simulink model "VectorTrackingSim"  (R2023a)
settings: Solver=FixedStepAuto  StartTime=Start_Time  StopTime=End_Time  FixedStep=Time_Step  RelTol=1e-3
values from neighbouring files (symbols this model uses):
  BSFC_LUT = aircraft.BSFC_LUT    [FVDM_Noise.m]    (also in FVDM_Truth.m)
  STGeometry = aircraft.STGeometry    [FVDM_Noise.m]    (also in FVDM_Truth.m)
  Vehicle = aircraft.Vehicle    [FVDM_Noise.m]    (also in FVDM_Truth.m)
undefined symbols (not defined in the file or in its folder): dayofyear, Earth, Initial_X, lookaheadDist, PowerFactor_LUT, waypoints, WGS84
libraries: slpidlib x7, simulink_extras x3, aerolibtransform2 x1, aerolibatmos2 x1, uavalgslib x1
(part 1 of 2)
settings Model: Creator=izc0018  LastModifiedBy=noahm
settings DebuggingCC: AlgebraicLoopMsg=none  UnconnectedInputMsg=warning  UnconnectedOutputMsg=warning  UnconnectedLineMsg=warning
settings HardwareCC: ProdBitPerLong=64  ProdLargestAtomicFloat=None  ProdHWDeviceType=AMD->Athlon 64
settings ModelReferenceCC: EnableRefExpFcnMdlSchedulingChecks=on  ModelReferenceMinAlgLoopOccurrences=on
settings RTWCC: DLArmComputeVersion=19.05

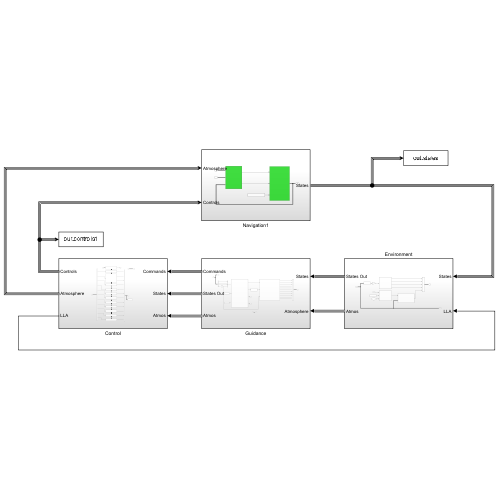
[thumbnail: Simulink's stored preview of the top-level diagram]
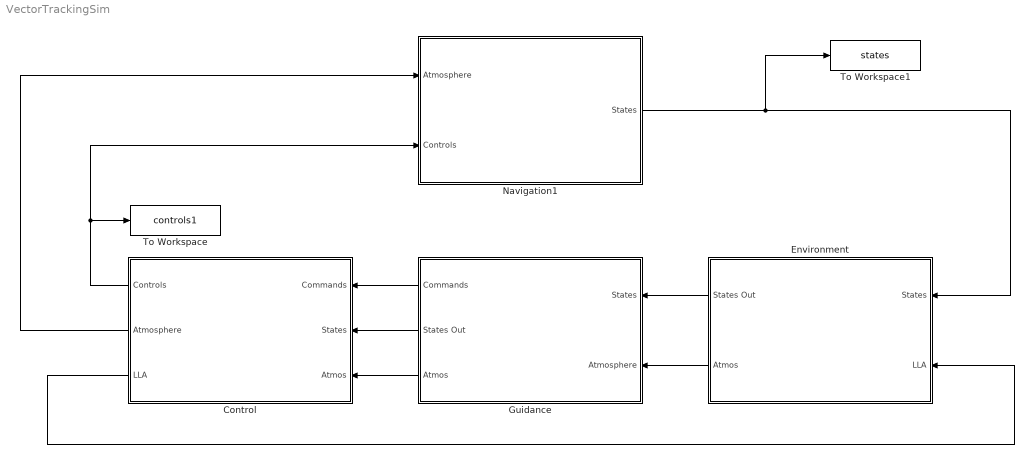
== system VectorTrackingSim ==
  Control : Subsystem
  Environment : Subsystem
  Guidance : Subsystem
  Navigation1 : Subsystem
  To Workspace : ToWorkspace  VariableName=controls1  SampleTime=-1
      settings: Save2DSignal=2-D array (concatenate along first dimension)
  To Workspace1 : ToWorkspace  VariableName=states  SampleTime=-1
      settings: Save2DSignal=2-D array (concatenate along first dimension)
  wires:
  Control/2(Atmosphere) -> Navigation1/1(Atmosphere)
  Guidance/1(Commands) -> Control/1(Commands)
  Environment/2(Atmos) -> Guidance/2(Atmosphere)
  Navigation1/1(States) -> To Workspace1/1, Environment/1(States)
  Control/3(LLA) -> Environment/2(LLA)
  Guidance/2(States Out) -> Control/2(States)
  Guidance/3(Atmos) -> Control/3(Atmos)
  Control/1(Controls) -> Navigation1/2(Controls), To Workspace/1
  Environment/1(States Out) -> Guidance/1(States)

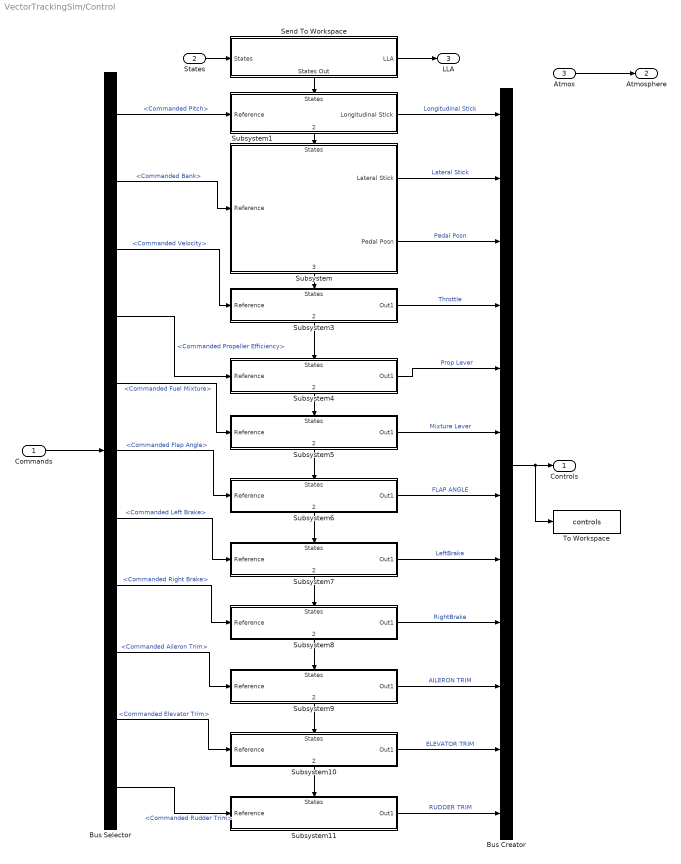
== system VectorTrackingSim/Control ==
  Commands : Inport
  States : Inport  Port=2
  Atmos : Inport  Port=3
  Bus Creator : BusCreator  Inputs=12
  Bus Selector : BusSelector  OutputSignals=Commanded Pitch,Commanded Bank,Commanded Velocity,Commanded Propeller Efficiency,Commanded Fuel Mixture,Commanded Flap Angle,Commanded Left Brake,Commanded Right Brake,Commanded Aileron Trim,Commanded Elevator Trim,Commanded Rudder Trim
  Send To Workspace : Subsystem
      settings: PortSchema="{\"entries\":[{\"content\":{\"sides\":[{\"content\":{\"connectorIds\":[\"In1\"]},\"type\":\"ConnectorPlacement.EquallySpacedRectSide\",\"uuid\":\"f8d70518-feba-4467-9144-e72499141e10\"},{\"content\":{\"connectorIds\":[\"Out1\"],\"side\":\"RIGHT\"},\"type\":\"ConnectorPlacement.EquallySpacedRectSide\",\"uuid\":\"0d837ca8-6650-40ee-933a-3521e14176de\"},{\"content\":{\"side\":\"TOP\"},\"type\":\"ConnectorPlacement.EquallySpacedRectSide\",\"uuid\":\"54f7b60b-7724-46f0-8f38-219401d515c7\"},{\"content\":{\"connectorIds\":[\"Out2\"],\"side\":\"BOTTOM\"},\"type\":\"ConnectorPlacement.EquallySpacedRectSide\",\"uuid\":\"f1e71b5c-4796-4085-9245-75f71ccb39d6\"}]},\"type\":\"ConnectorPlacement.EquallySpacedConnector\",\"uuid\":\"946e06f8-2adb-45c5-9153-0b4b2f8d0bb6\"}],\"packageUris\":[\"http://schema.mathworks.com/mf0/Connector/R2020b\"],\"version\":\"1.0\"}"
  Subsystem : Subsystem
      settings: PortSchema="{\"entries\":[{\"content\":{\"sides\":[{\"content\":{\"connectorIds\":[\"In1\"]},\"type\":\"ConnectorPlacement.EquallySpacedRectSide\",\"uuid\":\"5ea7349d-baf6-49c5-809d-4b912ce56d76\"},{\"content\":{\"connectorIds\":[\"Out1\",\"Out2\"],\"side\":\"RIGHT\"},\"type\":\"ConnectorPlacement.EquallySpacedRectSide\",\"uuid\":\"ab3ceec7-e245-42b0-9eb8-e3a68951e219\"},{\"content\":{\"connectorIds\":[\"In2\"],\"side\":\"TOP\"},\"type\":\"ConnectorPlacement.EquallySpacedRectSide\",\"uuid\":\"18178c43-0035-4aec-a3ba-011af3830f5c\"},{\"content\":{\"connectorIds\":[\"Out3\"],\"side\":\"BOTTOM\"},\"type\":\"ConnectorPlacement.EquallySpacedRectSide\",\"uuid\":\"88476787-2df8-4308-98f2-16231590cef9\"}]},\"type\":\"ConnectorPlacement.EquallySpacedConnector\",\"uuid\":\"0f7476f8-a4e6-4d2f-9698-249fd1b1cc90\"}],\"packageUris\":[\"http://schema.mathworks.com/mf0/Connector/R2020b\"],\"version\":\"1.0\"}"
  Subsystem1 : Subsystem
      settings: PortSchema="{\"entries\":[{\"content\":{\"sides\":[{\"content\":{\"connectorIds\":[\"In1\"]},\"type\":\"ConnectorPlacement.EquallySpacedRectSide\",\"uuid\":\"df1e81ab-d97f-43f0-8cd1-ba06c25288e8\"},{\"content\":{\"connectorIds\":[\"Out1\"],\"side\":\"RIGHT\"},\"type\":\"ConnectorPlacement.EquallySpacedRectSide\",\"uuid\":\"fe7f65be-8a13-42ab-8ffa-afe418a633fa\"},{\"content\":{\"connectorIds\":[\"In2\"],\"side\":\"TOP\"},\"type\":\"ConnectorPlacement.EquallySpacedRectSide\",\"uuid\":\"4762097a-1dfd-4646-aeb3-678774417eb9\"},{\"content\":{\"connectorIds\":[\"Out2\"],\"side\":\"BOTTOM\"},\"type\":\"ConnectorPlacement.EquallySpacedRectSide\",\"uuid\":\"338e28fc-4594-4f48-8379-f1c16de78061\"}]},\"type\":\"ConnectorPlacement.EquallySpacedConnector\",\"uuid\":\"e1e6a329-5243-44ef-b6a4-a2802fff17f2\"}],\"packageUris\":[\"http://schema.mathworks.com/mf0/Connector/R2020b\"],\"version\":\"1.0\"}"
  Subsystem10 : Subsystem
      settings: PortSchema="{\"entries\":[{\"content\":{\"sides\":[{\"content\":{\"connectorIds\":[\"In1\"]},\"type\":\"ConnectorPlacement.EquallySpacedRectSide\",\"uuid\":\"df1e81ab-d97f-43f0-8cd1-ba06c25288e8\"},{\"content\":{\"connectorIds\":[\"Out1\"],\"side\":\"RIGHT\"},\"type\":\"ConnectorPlacement.EquallySpacedRectSide\",\"uuid\":\"fe7f65be-8a13-42ab-8ffa-afe418a633fa\"},{\"content\":{\"connectorIds\":[\"In2\"],\"side\":\"TOP\"},\"type\":\"ConnectorPlacement.EquallySpacedRectSide\",\"uuid\":\"4762097a-1dfd-4646-aeb3-678774417eb9\"},{\"content\":{\"connectorIds\":[\"Out2\"],\"side\":\"BOTTOM\"},\"type\":\"ConnectorPlacement.EquallySpacedRectSide\",\"uuid\":\"ca232b1a-28ac-4e7a-b8a6-76103b2c6113\"}]},\"type\":\"ConnectorPlacement.EquallySpacedConnector\",\"uuid\":\"e1e6a329-5243-44ef-b6a4-a2802fff17f2\"}],\"packageUris\":[\"http://schema.mathworks.com/mf0/Connector/R2020b\"],\"version\":\"1.0\"}"
  Subsystem11 : Subsystem
      settings: PortSchema="{\"entries\":[{\"content\":{\"sides\":[{\"content\":{\"connectorIds\":[\"In1\"]},\"type\":\"ConnectorPlacement.EquallySpacedRectSide\",\"uuid\":\"df1e81ab-d97f-43f0-8cd1-ba06c25288e8\"},{\"content\":{\"connectorIds\":[\"Out1\"],\"side\":\"RIGHT\"},\"type\":\"ConnectorPlacement.EquallySpacedRectSide\",\"uuid\":\"fe7f65be-8a13-42ab-8ffa-afe418a633fa\"},{\"content\":{\"connectorIds\":[\"In2\"],\"side\":\"TOP\"},\"type\":\"ConnectorPlacement.EquallySpacedRectSide\",\"uuid\":\"4762097a-1dfd-4646-aeb3-678774417eb9\"}]},\"type\":\"ConnectorPlacement.EquallySpacedConnector\",\"uuid\":\"e1e6a329-5243-44ef-b6a4-a2802fff17f2\"}],\"packageUris\":[\"http://schema.mathworks.com/mf0/Connector/R2020b\"],\"version\":\"1.0\"}"
  Subsystem3 : Subsystem
      settings: PortSchema="{\"entries\":[{\"content\":{\"sides\":[{\"content\":{\"connectorIds\":[\"In1\"]},\"type\":\"ConnectorPlacement.EquallySpacedRectSide\",\"uuid\":\"df1e81ab-d97f-43f0-8cd1-ba06c25288e8\"},{\"content\":{\"connectorIds\":[\"Out1\"],\"side\":\"RIGHT\"},\"type\":\"ConnectorPlacement.EquallySpacedRectSide\",\"uuid\":\"fe7f65be-8a13-42ab-8ffa-afe418a633fa\"},{\"content\":{\"connectorIds\":[\"In2\"],\"side\":\"TOP\"},\"type\":\"ConnectorPlacement.EquallySpacedRectSide\",\"uuid\":\"4762097a-1dfd-4646-aeb3-678774417eb9\"},{\"content\":{\"connectorIds\":[\"Out2\"],\"side\":\"BOTTOM\"},\"type\":\"ConnectorPlacement.EquallySpacedRectSide\",\"uuid\":\"eb7acd08-7b98-4b28-a61a-3ca4385205ec\"}]},\"type\":\"ConnectorPlacement.EquallySpacedConnector\",\"uuid\":\"e1e6a329-5243-44ef-b6a4-a2802fff17f2\"}],\"packageUris\":[\"http://schema.mathworks.com/mf0/Connector/R2020b\"],\"version\":\"1.0\"}"
  Subsystem4 : Subsystem
      settings: PortSchema="{\"entries\":[{\"content\":{\"sides\":[{\"content\":{\"connectorIds\":[\"In1\"]},\"type\":\"ConnectorPlacement.EquallySpacedRectSide\",\"uuid\":\"df1e81ab-d97f-43f0-8cd1-ba06c25288e8\"},{\"content\":{\"connectorIds\":[\"Out1\"],\"side\":\"RIGHT\"},\"type\":\"ConnectorPlacement.EquallySpacedRectSide\",\"uuid\":\"fe7f65be-8a13-42ab-8ffa-afe418a633fa\"},{\"content\":{\"connectorIds\":[\"In2\"],\"side\":\"TOP\"},\"type\":\"ConnectorPlacement.EquallySpacedRectSide\",\"uuid\":\"4762097a-1dfd-4646-aeb3-678774417eb9\"},{\"content\":{\"connectorIds\":[\"Out2\"],\"side\":\"BOTTOM\"},\"type\":\"ConnectorPlacement.EquallySpacedRectSide\",\"uuid\":\"aca1bd27-9370-4c71-9435-0c269f9a438b\"}]},\"type\":\"ConnectorPlacement.EquallySpacedConnector\",\"uuid\":\"e1e6a329-5243-44ef-b6a4-a2802fff17f2\"}],\"packageUris\":[\"http://schema.mathworks.com/mf0/Connector/R2020b\"],\"version\":\"1.0\"}"
  Subsystem5 : Subsystem
      settings: PortSchema="{\"entries\":[{\"content\":{\"sides\":[{\"content\":{\"connectorIds\":[\"In1\"]},\"type\":\"ConnectorPlacement.EquallySpacedRectSide\",\"uuid\":\"df1e81ab-d97f-43f0-8cd1-ba06c25288e8\"},{\"content\":{\"connectorIds\":[\"Out1\"],\"side\":\"RIGHT\"},\"type\":\"ConnectorPlacement.EquallySpacedRectSide\",\"uuid\":\"fe7f65be-8a13-42ab-8ffa-afe418a633fa\"},{\"content\":{\"connectorIds\":[\"In2\"],\"side\":\"TOP\"},\"type\":\"ConnectorPlacement.EquallySpacedRectSide\",\"uuid\":\"4762097a-1dfd-4646-aeb3-678774417eb9\"},{\"content\":{\"connectorIds\":[\"Out2\"],\"side\":\"BOTTOM\"},\"type\":\"ConnectorPlacement.EquallySpacedRectSide\",\"uuid\":\"e3132084-5e8e-4693-9249-2c258902bcf1\"}]},\"type\":\"ConnectorPlacement.EquallySpacedConnector\",\"uuid\":\"e1e6a329-5243-44ef-b6a4-a2802fff17f2\"}],\"packageUris\":[\"http://schema.mathworks.com/mf0/Connector/R2020b\"],\"version\":\"1.0\"}"
  Subsystem6 : Subsystem
      settings: PortSchema="{\"entries\":[{\"content\":{\"sides\":[{\"content\":{\"connectorIds\":[\"In1\"]},\"type\":\"ConnectorPlacement.EquallySpacedRectSide\",\"uuid\":\"df1e81ab-d97f-43f0-8cd1-ba06c25288e8\"},{\"content\":{\"connectorIds\":[\"Out1\"],\"side\":\"RIGHT\"},\"type\":\"ConnectorPlacement.EquallySpacedRectSide\",\"uuid\":\"fe7f65be-8a13-42ab-8ffa-afe418a633fa\"},{\"content\":{\"connectorIds\":[\"In2\"],\"side\":\"TOP\"},\"type\":\"ConnectorPlacement.EquallySpacedRectSide\",\"uuid\":\"4762097a-1dfd-4646-aeb3-678774417eb9\"},{\"content\":{\"connectorIds\":[\"Out2\"],\"side\":\"BOTTOM\"},\"type\":\"ConnectorPlacement.EquallySpacedRectSide\",\"uuid\":\"44b8b4cf-3de4-40e9-9bc3-b7b2ed15b9c4\"}]},\"type\":\"ConnectorPlacement.EquallySpacedConnector\",\"uuid\":\"e1e6a329-5243-44ef-b6a4-a2802fff17f2\"}],\"packageUris\":[\"http://schema.mathworks.com/mf0/Connector/R2020b\"],\"version\":\"1.0\"}"
  Subsystem7 : Subsystem
      settings: PortSchema="{\"entries\":[{\"content\":{\"sides\":[{\"content\":{\"connectorIds\":[\"In1\"]},\"type\":\"ConnectorPlacement.EquallySpacedRectSide\",\"uuid\":\"df1e81ab-d97f-43f0-8cd1-ba06c25288e8\"},{\"content\":{\"connectorIds\":[\"Out1\"],\"side\":\"RIGHT\"},\"type\":\"ConnectorPlacement.EquallySpacedRectSide\",\"uuid\":\"fe7f65be-8a13-42ab-8ffa-afe418a633fa\"},{\"content\":{\"connectorIds\":[\"In2\"],\"side\":\"TOP\"},\"type\":\"ConnectorPlacement.EquallySpacedRectSide\",\"uuid\":\"4762097a-1dfd-4646-aeb3-678774417eb9\"},{\"content\":{\"connectorIds\":[\"Out2\"],\"side\":\"BOTTOM\"},\"type\":\"ConnectorPlacement.EquallySpacedRectSide\",\"uuid\":\"4aea28e3-05ae-492c-9523-17787d8052fd\"}]},\"type\":\"ConnectorPlacement.EquallySpacedConnector\",\"uuid\":\"e1e6a329-5243-44ef-b6a4-a2802fff17f2\"}],\"packageUris\":[\"http://schema.mathworks.com/mf0/Connector/R2020b\"],\"version\":\"1.0\"}"
  Subsystem8 : Subsystem
      settings: PortSchema="{\"entries\":[{\"content\":{\"sides\":[{\"content\":{\"connectorIds\":[\"In1\"]},\"type\":\"ConnectorPlacement.EquallySpacedRectSide\",\"uuid\":\"df1e81ab-d97f-43f0-8cd1-ba06c25288e8\"},{\"content\":{\"connectorIds\":[\"Out1\"],\"side\":\"RIGHT\"},\"type\":\"ConnectorPlacement.EquallySpacedRectSide\",\"uuid\":\"fe7f65be-8a13-42ab-8ffa-afe418a633fa\"},{\"content\":{\"connectorIds\":[\"In2\"],\"side\":\"TOP\"},\"type\":\"ConnectorPlacement.EquallySpacedRectSide\",\"uuid\":\"4762097a-1dfd-4646-aeb3-678774417eb9\"},{\"content\":{\"connectorIds\":[\"Out2\"],\"side\":\"BOTTOM\"},\"type\":\"ConnectorPlacement.EquallySpacedRectSide\",\"uuid\":\"60b425fe-182c-41c2-bc4c-aa97cb3d7ccf\"}]},\"type\":\"ConnectorPlacement.EquallySpacedConnector\",\"uuid\":\"e1e6a329-5243-44ef-b6a4-a2802fff17f2\"}],\"packageUris\":[\"http://schema.mathworks.com/mf0/Connector/R2020b\"],\"version\":\"1.0\"}"
  Subsystem9 : Subsystem
      settings: PortSchema="{\"entries\":[{\"content\":{\"sides\":[{\"content\":{\"connectorIds\":[\"In1\"]},\"type\":\"ConnectorPlacement.EquallySpacedRectSide\",\"uuid\":\"df1e81ab-d97f-43f0-8cd1-ba06c25288e8\"},{\"content\":{\"connectorIds\":[\"Out1\"],\"side\":\"RIGHT\"},\"type\":\"ConnectorPlacement.EquallySpacedRectSide\",\"uuid\":\"fe7f65be-8a13-42ab-8ffa-afe418a633fa\"},{\"content\":{\"connectorIds\":[\"In2\"],\"side\":\"TOP\"},\"type\":\"ConnectorPlacement.EquallySpacedRectSide\",\"uuid\":\"4762097a-1dfd-4646-aeb3-678774417eb9\"},{\"content\":{\"connectorIds\":[\"Out2\"],\"side\":\"BOTTOM\"},\"type\":\"ConnectorPlacement.EquallySpacedRectSide\",\"uuid\":\"88e2b07d-9cf7-412b-8368-04827ebf702b\"}]},\"type\":\"ConnectorPlacement.EquallySpacedConnector\",\"uuid\":\"e1e6a329-5243-44ef-b6a4-a2802fff17f2\"}],\"packageUris\":[\"http://schema.mathworks.com/mf0/Connector/R2020b\"],\"version\":\"1.0\"}"
  To Workspace : ToWorkspace  VariableName=controls  SampleTime=-1
      settings: Save2DSignal=2-D array (concatenate along first dimension)
  Controls : Outport
  Atmosphere : Outport  Port=2
  LLA : Outport  Port=3
  wires:
  Subsystem11/1(Out1) -> Bus Creator/12  "RUDDER TRIM"
  Subsystem9/1(Out1) -> Bus Creator/10  "AILERON TRIM"
  Subsystem1/1(Longitudinal Stick) -> Bus Creator/1  "Longitudinal Stick"
  Subsystem/1(Lateral Stick) -> Bus Creator/2  "Lateral Stick"
  Subsystem6/1(Out1) -> Bus Creator/7  "FLAP ANGLE"
  Subsystem5/1(Out1) -> Bus Creator/6  "Mixture Lever"
  Subsystem3/1(Out1) -> Bus Creator/4  "Throttle"
  Subsystem8/1(Out1) -> Bus Creator/9  "RightBrake"
  Subsystem/2(Pedal Posn) -> Bus Creator/3  "Pedal Posn"
  Subsystem4/1(Out1) -> Bus Creator/5  "Prop Lever"
  Subsystem7/1(Out1) -> Bus Creator/8  "LeftBrake"
  Subsystem10/1(Out1) -> Bus Creator/11  "ELEVATOR TRIM"
  Bus Creator/1 -> To Workspace/1, Controls/1
  Commands/1 -> Bus Selector/1
  Bus Selector/11 -> Subsystem11/1(Reference)  "<Commanded Rudder Trim>"
  Bus Selector/10 -> Subsystem10/1(Reference)  "<Commanded Elevator Trim>"
  Bus Selector/9 -> Subsystem9/1(Reference)  "<Commanded Aileron Trim>"
  Bus Selector/8 -> Subsystem8/1(Reference)  "<Commanded Right Brake>"
  Bus Selector/7 -> Subsystem7/1(Reference)  "<Commanded Left Brake>"
  Bus Selector/6 -> Subsystem6/1(Reference)  "<Commanded Flap Angle>"
  Bus Selector/5 -> Subsystem5/1(Reference)  "<Commanded Fuel Mixture>"
  Bus Selector/4 -> Subsystem4/1(Reference)  "<Commanded Propeller Efficiency>"
  Bus Selector/3 -> Subsystem3/1(Reference)  "<Commanded Velocity>"
  Bus Selector/1 -> Subsystem1/1(Reference)  "<Commanded Pitch>"
  Bus Selector/2 -> Subsystem/1(Reference)  "<Commanded Bank>"
  States/1 -> Send To Workspace/1(States)
  Send To Workspace/2(States Out) -> Subsystem1/2(States)
  Subsystem6/2(" ") -> Subsystem7/2(States)
  Subsystem9/2(" ") -> Subsystem10/2(States)
  Subsystem3/2(" ") -> Subsystem4/2(States)
  Subsystem/3(" ") -> Subsystem3/2(States)
  Subsystem1/2(" ") -> Subsystem/2(States)
  Subsystem7/2(" ") -> Subsystem8/2(States)
  Subsystem8/2(" ") -> Subsystem9/2(States)
  Subsystem5/2(" ") -> Subsystem6/2(States)
  Subsystem4/2(" ") -> Subsystem5/2(States)
  Subsystem10/2(" ") -> Subsystem11/2(States)
  Atmos/1 -> Atmosphere/1
  Send To Workspace/1(LLA) -> LLA/1

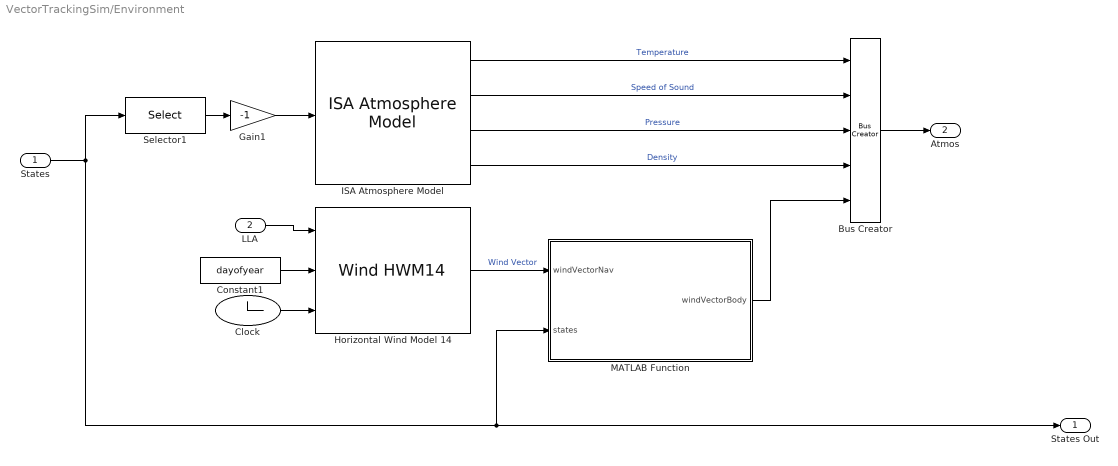
== system VectorTrackingSim/Environment ==
  States : Inport
  LLA : Inport  Port=2
  Bus Creator : BusCreator  Inputs=5
  Clock : Clock
  Constant1 : Constant  Value=dayofyear
  Gain1 : Gain  Gain=-1
  Horizontal Wind Model 14 : WindHWM14
  ISA Atmosphere Model : aerolibatmos2/ISA Atmosphere Model  custom=off  g=9.80665  gamma=1.4  R=287.0531  L=0.0065  h_trop=11000  h_strat=20000  rho0=1.225  P0=101325  T0=288.15  h0=0
  MATLAB Function : MATLAB Function  TreatAsAtomicUnit=on
  Selector1 : Selector  InputPortWidth=12  IndexOptions=Index vector (dialog)  Indices=[9]  OutputSizes=1
  States Out : Outport
  Atmos : Outport  Port=2
  wires:
  States/1 -> MATLAB Function/2(states), States Out/1, Selector1/1
  Selector1/1 -> Gain1/1
  ISA Atmosphere Model/2 -> Bus Creator/2  "Speed of Sound"
  ISA Atmosphere Model/3 -> Bus Creator/3  "Pressure"
  Bus Creator/1 -> Atmos/1
  ISA Atmosphere Model/1 -> Bus Creator/1  "Temperature"
  Gain1/1 -> ISA Atmosphere Model/1
  ISA Atmosphere Model/4 -> Bus Creator/4  "Density"
  LLA/1 -> Horizontal Wind Model 14/1
  Clock/1 -> Horizontal Wind Model 14/3
  Constant1/1 -> Horizontal Wind Model 14/2
  Horizontal Wind Model 14/1 -> MATLAB Function/1(windVectorNav)  "Wind Vector"
  MATLAB Function/1(windVectorBody) -> Bus Creator/5

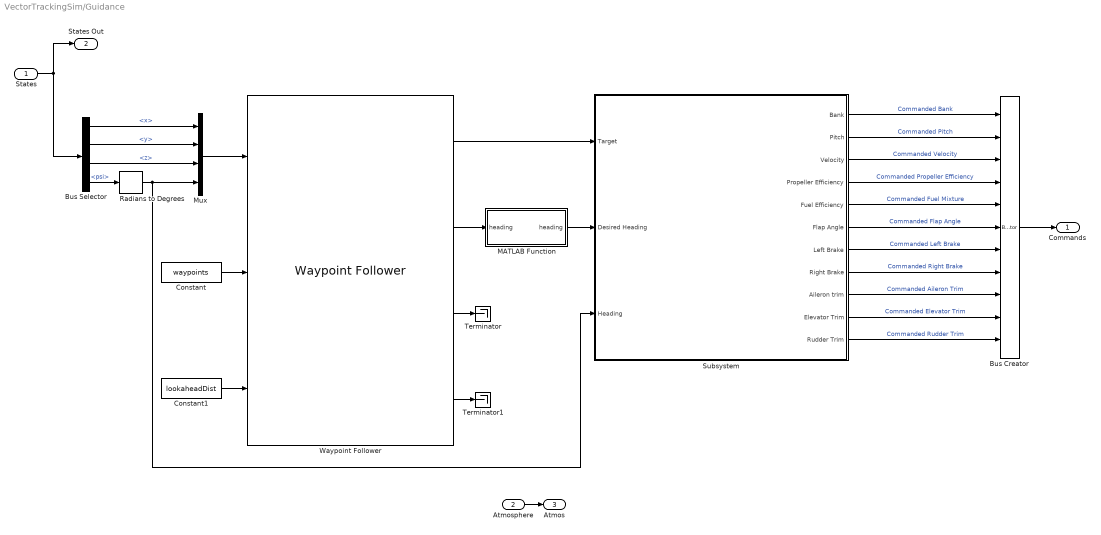
== system VectorTrackingSim/Guidance ==
  States : Inport
  Atmosphere : Inport  Port=2
  Bus Creator : BusCreator  Inputs=11
  Bus Selector : BusSelector  OutputSignals=x,y,z,psi
  Constant : Constant  Value=waypoints
  Constant1 : Constant  Value=lookaheadDist
  MATLAB Function : MATLAB Function  TreatAsAtomicUnit=on
  Mux : Mux
  Radians to Degrees : simulink_extras/Transformations/Radians to Degrees
  Subsystem : Subsystem
  Terminator : Terminator
  Terminator1 : Terminator
  Waypoint Follower : uavalgslib/Waypoint Follower  UAVType=fixed-wing  StartFrom=first  TransitionRadiusSource=internal  TransitionRadius=10  MinLookaheadDistance=0.1  YawInput=off  ShowCrossTrackErrorOutput=off  ShowStatusOutput=off  SimulateUsing=Code generation
  Commands : Outport
  States Out : Outport  Port=2
  Atmos : Outport  Port=3
  wires:
  Bus Creator/1 -> Commands/1
  Subsystem/1(Bank) -> Bus Creator/1  "Commanded Bank"
  Subsystem/2(Pitch) -> Bus Creator/2  "Commanded Pitch"
  Subsystem/3(Velocity) -> Bus Creator/3  "Commanded Velocity"
  Subsystem/4(Propeller Efficiency) -> Bus Creator/4  "Commanded Propeller Efficiency"
  Subsystem/5(Fuel Efficiency) -> Bus Creator/5  "Commanded Fuel Mixture"
  Subsystem/6(Flap Angle) -> Bus Creator/6  "Commanded Flap Angle"
  Subsystem/7(Left Brake) -> Bus Creator/7  "Commanded Left Brake"
  Subsystem/8(Right Brake) -> Bus Creator/8  "Commanded Right Brake"
  Subsystem/9(Aileron trim) -> Bus Creator/9  "Commanded Aileron Trim"
  Subsystem/10(Elevator Trim) -> Bus Creator/10  "Commanded Elevator Trim"
  Subsystem/11(Rudder Trim) -> Bus Creator/11  "Commanded Rudder Trim"
  States/1 -> Bus Selector/1, States Out/1
  Waypoint Follower/3 -> Terminator/1
  Waypoint Follower/4 -> Terminator1/1
  Constant/1 -> Waypoint Follower/2
  Constant1/1 -> Waypoint Follower/3
  Mux/1 -> Waypoint Follower/1
  Bus Selector/1 -> Mux/1  "<x>"
  Bus Selector/2 -> Mux/2  "<y>"
  Bus Selector/3 -> Mux/3  "<z>"
  Waypoint Follower/2 -> MATLAB Function/1("heading ")
  Atmosphere/1 -> Atmos/1
  Waypoint Follower/1 -> Subsystem/1(Target)
  MATLAB Function/1(heading) -> Subsystem/2(Desired Heading)
  Radians to Degrees/1 -> Mux/4, Subsystem/3(Heading)
  Bus Selector/4 -> Radians to Degrees/1  "<psi>"

== system VectorTrackingSim/Navigation1 ==
  Atmosphere : Inport
  Controls : Inport  Port=2
  Constant1 : Constant  Value=Vehicle.MassProp.Mass
  DA-40 Equations of Motion : Subsystem
  Flight Mechanics and Systems Models : Subsystem
  States : Outport
  wires:
  Flight Mechanics and Systems Models/1(Fb) -> DA-40 Equations of Motion/1(Fb [lb])
  Flight Mechanics and Systems Models/2(Mb) -> DA-40 Equations of Motion/2(Mb [lb-ft])
  Controls/1 -> Flight Mechanics and Systems Models/2(Control Commands)
  Atmosphere/1 -> Flight Mechanics and Systems Models/1(Atmosphere)
  Constant1/1 -> DA-40 Equations of Motion/3(Mass Properties)
  DA-40 Equations of Motion/1(States) -> Flight Mechanics and Systems Models/3(States), States/1

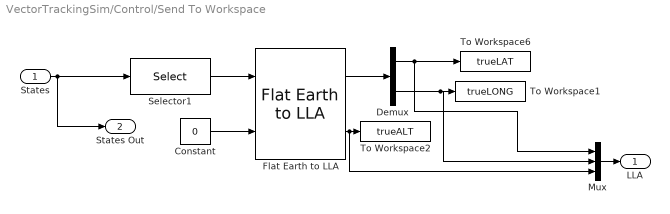
== system VectorTrackingSim/Control/Send To Workspace ==
  States : Inport
  Constant : Constant  Value=0
  Demux : Demux  Outputs=2
  Flat Earth to LLA : aerolibtransform2/Flat Earth to LLA  units=Metric (MKS)  ptype=Earth (WGS84)  F=1/298.257223563  R=6378137  refPosPort=off  LL0=refLLA  psi=0
  Mux : Mux  Inputs=3
  Selector1 : Selector  InputPortWidth=12  IndexOptions=Index vector (dialog)  Indices=[7:9]  OutputSizes=1
  To Workspace1 : ToWorkspace  VariableName=trueLONG  SampleTime=-1
  To Workspace2 : ToWorkspace  VariableName=trueALT  SampleTime=-1
  To Workspace6 : ToWorkspace  VariableName=trueLAT  SampleTime=-1
  LLA : Outport
  States Out : Outport  Port=2
  wires:
  States/1 -> States Out/1, Selector1/1
  Selector1/1 -> Flat Earth to LLA/1
  Constant/1 -> Flat Earth to LLA/2
  Flat Earth to LLA/2 -> Mux/3, To Workspace2/1
  Flat Earth to LLA/1 -> Demux/1
  Demux/1 -> Mux/1, To Workspace6/1
  Demux/2 -> Mux/2, To Workspace1/1
  Mux/1 -> LLA/1

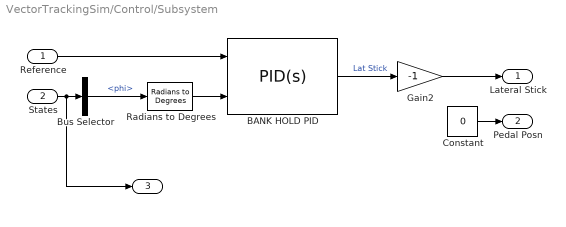
== system VectorTrackingSim/Control/Subsystem ==
  Reference : Inport
  States : Inport  Port=2
  BANK HOLD PID : slpidlib/PID Controller (2DOF)  Controller=PID  Form=Parallel  TimeDomain=Continuous-time  UseExternalTs=off  SampleTime=-1  IntegratorMethod=Forward Euler  FilterMethod=Forward Euler  ControllerParametersSource=internal  P=0.107891692261891  I=0.133343747084316  UseKiTs=off  D=0.0171409705451499  N=25.8919437213056  UseFilter=on  b=0.548332573243903  c=0.00478750158934923  TunerSelectOption=Transfer Function Based (PID Tuner App)  InitialConditionSource=internal  InitialConditionForIntegrator=0  InitialConditionForFilter=0  DifferentiatorICPrevScaledInput=0  ExternalReset=none  TrackingMode=off  Kt=1  LimitOutput=on  SatLimitsSource=internal  UpperSaturationLimit=1  LowerSaturationLimit=-1  LinearizeAsGain=on  AntiWindupMode=clamping  Kb=1  LimitIntegrator=off  UpperIntegratorSaturationLimit=inf  LowerIntegratorSaturationLimit=-inf  POutMin=[]  POutMax=[]  IOutMin=[]  IOutMax=[]  DOutMin=[]  DOutMax=[]  NOutMin=[]  NOutMax=[]  bOutMin=[]  bOutMax=[]  cOutMin=[]  cOutMax=[]  SumOutMin=[]  SumOutMax=[]  SaturationOutMin=[]  SaturationOutMax=[]  PParamMin=[]  PParamMax=[]  IParamMin=[]  IParamMax=[]  DParamMin=[]  DParamMax=[]  NParamMin=[]  NParamMax=[]  bParamMin=[]  bParamMax=[]  cParamMin=[]  cParamMax=[]  KbParamMin=[]  KbParamMax=[]  KtParamMin=[]  KtParamMax=[]  KbOutMin=[]  KbOutMax=[]  KtOutMin=[]  KtOutMax=[]  IntegratorOutMin=[]  IntegratorOutMax=[]  FilterOutMin=[]  FilterOutMax=[]  SumI1OutMin=[]  SumI1OutMax=[]  SumI2OutMin=[]  SumI2OutMax=[]  SumI3OutMin=[]  SumI3OutMax=[]  SumI4OutMin=[]  SumI4OutMax=[]  SumDOutMin=[]  SumDOutMax=[]  Sum1OutMin=[]  Sum1OutMax=[]  Sum2OutMin=[]  Sum2OutMax=[]  Sum3OutMin=[]  Sum3OutMax=[]  DifferentiatorOutMin=[]  DifferentiatorOutMax=[]  FilterDiffOutCoefMin=[]  FilterDiffOutCoefMax=[]  ReciprocalOutMin=[]  ReciprocalOutMax=[]  SumDenOutMin=[]  SumDenOutMax=[]  SumNumOutMin=[]  SumNumOutMax=[]  DivideOutMin=[]  DivideOutMax=[]  UdiffTsProdOutMin=[]  UdiffTsProdOutMax=[]  NTsProdOutMin=[]  NTsProdOutMax=[]  UintegralTsProdOutMin=[]  UintegralTsProdOutMax=[]  UngainTsProdOutMin=[]  UngainTsProdOutMax=[]  ClampingZeroOutDataTypeStr=Inherit: Inherit via back propagation  ClampingZeroOutMin=[]  ClampingZeroOutMax=[]  FilterDenConstantOutDataTypeStr=Inherit: Inherit via back propagation  FilterDenConstantOutMin=[]  FilterDenConstantOutMax=[]  PCopyOutDataTypeStr=Inherit: Inherit via back propagation  PCopyOutMin=[]  PCopyOutMax=[]  NCopyOutDataTypeStr=Inherit: Inherit via back propagation  NCopyOutMin=[]  NCopyOutMax=[]  IntegratorContinuousStateAttributes=''  IntegratorStateMustResolveToSignalObject=off  IntegratorRTWStateStorageClass=Auto  FilterContinuousStateAttributes=''  FilterStateMustResolveToSignalObject=off  FilterRTWStateStorageClass=Auto  ParallelPVariant=InternalParameters  IdealPVariant=Disabled  IVariant=InternalParameters  DVariant=InternalParameters  bVariant=InternalParameters  cVariant=InternalParameters  IntegratorVariant=Continuous  SatVariant=Enabled  AWVariant=ContClampingParallel  PCopyVariant=Disabled  TRVariant=Disabled  FdbkBlocksVariant=Forward  IdealPFdbkVariant=Disabled  SatFdbkVariant=Disabled  DerivativeFilterVariant=ContFilter  NVariant=InternalParameters  NCopyVariant=Disabled  FilterICVariant=InternalICsFilter  IntegratorICVariant=InternalICs  ExternalResetVariant=Disabled  TRSumVariant=Passthrough  SumFdbkVariant=Disabled  SumVariant=Sum_PID  TsampFilterVariant=InternalTs  TsampNgainVariant=Passthrough  TsampIntegralVariant=Disabled_SignalSpec  ExternalSaturationOutDataTypeStr=Inherit: Same as second input
  Bus Selector : BusSelector  OutputSignals=phi
  Constant : Constant  Value=0
  Gain2 : Gain  Gain=-1
  Radians to Degrees : simulink_extras/Transformations/Radians to Degrees
  Lateral Stick : Outport
  Pedal Posn : Outport  Port=2
  " " : Outport  Port=3
  wires:
  BANK HOLD PID/1 -> Gain2/1  "Lat Stick"
  Gain2/1 -> Lateral Stick/1
  Radians to Degrees/1 -> BANK HOLD PID/2
  States/1 -> " "/1, Bus Selector/1
  Bus Selector/1 -> Radians to Degrees/1  "<phi>"
  Reference/1 -> BANK HOLD PID/1
  Constant/1 -> Pedal Posn/1

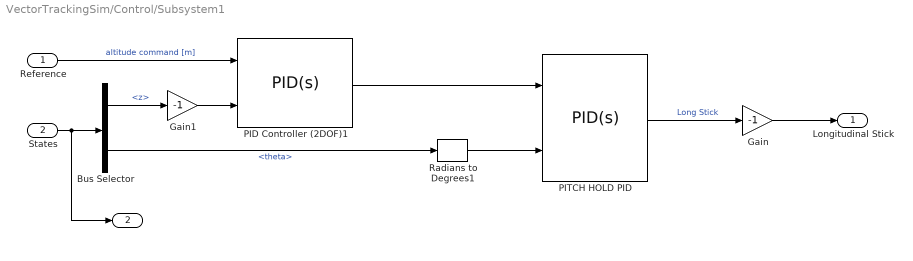
== system VectorTrackingSim/Control/Subsystem1 ==
  Reference : Inport
  States : Inport  Port=2
  Bus Selector : BusSelector  OutputSignals=z,theta
  Gain : Gain  Gain=-1
  Gain1 : Gain  Gain=-1
  PID Controller (2DOF)1 : slpidlib/PID Controller (2DOF)  Controller=PID  Form=Parallel  TimeDomain=Continuous-time  UseExternalTs=off  SampleTime=-1  IntegratorMethod=Forward Euler  FilterMethod=Forward Euler  ControllerParametersSource=internal  P=0.392178102036374  I=0.0013184227867295  UseKiTs=off  D=-0.0973934682361479  N=4.02673925817559  UseFilter=on  b=1  c=1  TunerSelectOption=Transfer Function Based (PID Tuner App)  InitialConditionSource=internal  InitialConditionForIntegrator=0  InitialConditionForFilter=0  DifferentiatorICPrevScaledInput=0  ExternalReset=none  TrackingMode=off  Kt=1  LimitOutput=on  SatLimitsSource=internal  UpperSaturationLimit=15  LowerSaturationLimit=-15  LinearizeAsGain=on  AntiWindupMode=clamping  Kb=1  LimitIntegrator=off  UpperIntegratorSaturationLimit=inf  LowerIntegratorSaturationLimit=-inf  POutMin=[]  POutMax=[]  IOutMin=[]  IOutMax=[]  DOutMin=[]  DOutMax=[]  NOutMin=[]  NOutMax=[]  bOutMin=[]  bOutMax=[]  cOutMin=[]  cOutMax=[]  SumOutMin=[]  SumOutMax=[]  SaturationOutMin=[]  SaturationOutMax=[]  PParamMin=[]  PParamMax=[]  IParamMin=[]  IParamMax=[]  DParamMin=[]  DParamMax=[]  NParamMin=[]  NParamMax=[]  bParamMin=[]  bParamMax=[]  cParamMin=[]  cParamMax=[]  KbParamMin=[]  KbParamMax=[]  KtParamMin=[]  KtParamMax=[]  KbOutMin=[]  KbOutMax=[]  KtOutMin=[]  KtOutMax=[]  IntegratorOutMin=[]  IntegratorOutMax=[]  FilterOutMin=[]  FilterOutMax=[]  SumI1OutMin=[]  SumI1OutMax=[]  SumI2OutMin=[]  SumI2OutMax=[]  SumI3OutMin=[]  SumI3OutMax=[]  SumI4OutMin=[]  SumI4OutMax=[]  SumDOutMin=[]  SumDOutMax=[]  Sum1OutMin=[]  Sum1OutMax=[]  Sum2OutMin=[]  Sum2OutMax=[]  Sum3OutMin=[]  Sum3OutMax=[]  DifferentiatorOutMin=[]  DifferentiatorOutMax=[]  FilterDiffOutCoefMin=[]  FilterDiffOutCoefMax=[]  ReciprocalOutMin=[]  ReciprocalOutMax=[]  SumDenOutMin=[]  SumDenOutMax=[]  SumNumOutMin=[]  SumNumOutMax=[]  DivideOutMin=[]  DivideOutMax=[]  UdiffTsProdOutMin=[]  UdiffTsProdOutMax=[]  NTsProdOutMin=[]  NTsProdOutMax=[]  UintegralTsProdOutMin=[]  UintegralTsProdOutMax=[]  UngainTsProdOutMin=[]  UngainTsProdOutMax=[]  ClampingZeroOutDataTypeStr=Inherit: Inherit via back propagation  ClampingZeroOutMin=[]  ClampingZeroOutMax=[]  FilterDenConstantOutDataTypeStr=Inherit: Inherit via back propagation  FilterDenConstantOutMin=[]  FilterDenConstantOutMax=[]  PCopyOutDataTypeStr=Inherit: Inherit via back propagation  PCopyOutMin=[]  PCopyOutMax=[]  NCopyOutDataTypeStr=Inherit: Inherit via back propagation  NCopyOutMin=[]  NCopyOutMax=[]  IntegratorContinuousStateAttributes=''  IntegratorStateMustResolveToSignalObject=off  IntegratorRTWStateStorageClass=Auto  FilterContinuousStateAttributes=''  FilterStateMustResolveToSignalObject=off  FilterRTWStateStorageClass=Auto  ParallelPVariant=InternalParameters  IdealPVariant=Disabled  IVariant=InternalParameters  DVariant=InternalParameters  bVariant=InternalParameters  cVariant=InternalParameters  IntegratorVariant=Continuous  SatVariant=Enabled  AWVariant=ContClampingParallel  PCopyVariant=Disabled  TRVariant=Disabled  FdbkBlocksVariant=Forward  IdealPFdbkVariant=Disabled  SatFdbkVariant=Disabled  DerivativeFilterVariant=ContFilter  NVariant=InternalParameters  NCopyVariant=Disabled  FilterICVariant=InternalICsFilter  IntegratorICVariant=InternalICs  ExternalResetVariant=Disabled  TRSumVariant=Passthrough  SumFdbkVariant=Disabled  SumVariant=Sum_PID  TsampFilterVariant=InternalTs  TsampNgainVariant=Passthrough  TsampIntegralVariant=Disabled_SignalSpec  ExternalSaturationOutDataTypeStr=Inherit: Same as second input
  PITCH HOLD PID : slpidlib/PID Controller (2DOF)  Controller=PID  Form=Parallel  TimeDomain=Continuous-time  UseExternalTs=off  SampleTime=-1  IntegratorMethod=Forward Euler  FilterMethod=Forward Euler  ControllerParametersSource=internal  P=0.06  I=0.01  UseKiTs=off  D=0.02  N=100  UseFilter=on  b=1  c=0  TunerSelectOption=Transfer Function Based (PID Tuner App)  InitialConditionSource=internal  InitialConditionForIntegrator=0  InitialConditionForFilter=0  DifferentiatorICPrevScaledInput=0  ExternalReset=none  TrackingMode=off  Kt=1  LimitOutput=on  SatLimitsSource=internal  UpperSaturationLimit=1  LowerSaturationLimit=-1  LinearizeAsGain=on  AntiWindupMode=clamping  Kb=1  LimitIntegrator=off  UpperIntegratorSaturationLimit=inf  LowerIntegratorSaturationLimit=-inf  POutMin=[]  POutMax=[]  IOutMin=[]  IOutMax=[]  DOutMin=[]  DOutMax=[]  NOutMin=[]  NOutMax=[]  bOutMin=[]  bOutMax=[]  cOutMin=[]  cOutMax=[]  SumOutMin=[]  SumOutMax=[]  SaturationOutMin=[]  SaturationOutMax=[]  PParamMin=[]  PParamMax=[]  IParamMin=[]  IParamMax=[]  DParamMin=[]  DParamMax=[]  NParamMin=[]  NParamMax=[]  bParamMin=[]  bParamMax=[]  cParamMin=[]  cParamMax=[]  KbParamMin=[]  KbParamMax=[]  KtParamMin=[]  KtParamMax=[]  KbOutMin=[]  KbOutMax=[]  KtOutMin=[]  KtOutMax=[]  IntegratorOutMin=[]  IntegratorOutMax=[]  FilterOutMin=[]  FilterOutMax=[]  SumI1OutMin=[]  SumI1OutMax=[]  SumI2OutMin=[]  SumI2OutMax=[]  SumI3OutMin=[]  SumI3OutMax=[]  SumI4OutMin=[]  SumI4OutMax=[]  SumDOutMin=[]  SumDOutMax=[]  Sum1OutMin=[]  Sum1OutMax=[]  Sum2OutMin=[]  Sum2OutMax=[]  Sum3OutMin=[]  Sum3OutMax=[]  DifferentiatorOutMin=[]  DifferentiatorOutMax=[]  FilterDiffOutCoefMin=[]  FilterDiffOutCoefMax=[]  ReciprocalOutMin=[]  ReciprocalOutMax=[]  SumDenOutMin=[]  SumDenOutMax=[]  SumNumOutMin=[]  SumNumOutMax=[]  DivideOutMin=[]  DivideOutMax=[]  UdiffTsProdOutMin=[]  UdiffTsProdOutMax=[]  NTsProdOutMin=[]  NTsProdOutMax=[]  UintegralTsProdOutMin=[]  UintegralTsProdOutMax=[]  UngainTsProdOutMin=[]  UngainTsProdOutMax=[]  ClampingZeroOutDataTypeStr=Inherit: Inherit via back propagation  ClampingZeroOutMin=[]  ClampingZeroOutMax=[]  FilterDenConstantOutDataTypeStr=Inherit: Inherit via back propagation  FilterDenConstantOutMin=[]  FilterDenConstantOutMax=[]  PCopyOutDataTypeStr=Inherit: Inherit via back propagation  PCopyOutMin=[]  PCopyOutMax=[]  NCopyOutDataTypeStr=Inherit: Inherit via back propagation  NCopyOutMin=[]  NCopyOutMax=[]  IntegratorContinuousStateAttributes=''  IntegratorStateMustResolveToSignalObject=off  IntegratorRTWStateStorageClass=Auto  FilterContinuousStateAttributes=''  FilterStateMustResolveToSignalObject=off  FilterRTWStateStorageClass=Auto  ParallelPVariant=InternalParameters  IdealPVariant=Disabled  IVariant=InternalParameters  DVariant=InternalParameters  bVariant=InternalParameters  cVariant=InternalParameters  IntegratorVariant=Continuous  SatVariant=Enabled  AWVariant=ContClampingParallel  PCopyVariant=Disabled  TRVariant=Disabled  FdbkBlocksVariant=Forward  IdealPFdbkVariant=Disabled  SatFdbkVariant=Disabled  DerivativeFilterVariant=ContFilter  NVariant=InternalParameters  NCopyVariant=Disabled  FilterICVariant=InternalICsFilter  IntegratorICVariant=InternalICs  ExternalResetVariant=Disabled  TRSumVariant=Passthrough  SumFdbkVariant=Disabled  SumVariant=Sum_PID  TsampFilterVariant=InternalTs  TsampNgainVariant=Passthrough  TsampIntegralVariant=Disabled_SignalSpec  ExternalSaturationOutDataTypeStr=Inherit: Same as second input
  Radians to Degrees1 : simulink_extras/Transformations/Radians to Degrees
  Longitudinal Stick : Outport
  " " : Outport  Port=2
  wires:
  PID Controller (2DOF)1/1 -> PITCH HOLD PID/1
  Reference/1 -> PID Controller (2DOF)1/1  "altitude command [m]"
  PITCH HOLD PID/1 -> Gain/1  "Long Stick"
  Radians to Degrees1/1 -> PITCH HOLD PID/2
  States/1 -> " "/1, Bus Selector/1
  Gain/1 -> Longitudinal Stick/1
  Gain1/1 -> PID Controller (2DOF)1/2
  Bus Selector/1 -> Gain1/1  "<z>"
  Bus Selector/2 -> Radians to Degrees1/1  "<theta>"

== system VectorTrackingSim/Control/Subsystem10 ==
  Reference : Inport
  States : Inport  Port=2
  Out1 : Outport
  " " : Outport  Port=2
  wires:
  Reference/1 -> Out1/1
  States/1 -> " "/1

== system VectorTrackingSim/Control/Subsystem11 ==
  Reference : Inport
  States : Inport  Port=2
  Terminator : Terminator
  Out1 : Outport
  wires:
  Reference/1 -> Out1/1
  States/1 -> Terminator/1

== system VectorTrackingSim/Control/Subsystem3 ==
  Reference : Inport
  States : Inport  Port=2
  MATLAB Function : MATLAB Function  TreatAsAtomicUnit=on
  PID Controller (2DOF) : slpidlib/PID Controller (2DOF)  Controller=PID  Form=Parallel  TimeDomain=Continuous-time  UseExternalTs=off  SampleTime=-1  IntegratorMethod=Forward Euler  FilterMethod=Forward Euler  ControllerParametersSource=internal  P=0.497904922106352  I=0.0979272469433752  UseKiTs=off  D=-0.183968459268293  N=2.70646894628946  UseFilter=on  b=0.574546090887085  c=0.574546090887085  TunerSelectOption=Transfer Function Based (PID Tuner App)  InitialConditionSource=internal  InitialConditionForIntegrator=0  InitialConditionForFilter=0  DifferentiatorICPrevScaledInput=0  ExternalReset=none  TrackingMode=off  Kt=1  LimitOutput=on  SatLimitsSource=internal  UpperSaturationLimit=1  LowerSaturationLimit=0  LinearizeAsGain=on  AntiWindupMode=none  Kb=1  LimitIntegrator=off  UpperIntegratorSaturationLimit=inf  LowerIntegratorSaturationLimit=-inf  POutMin=[]  POutMax=[]  IOutMin=[]  IOutMax=[]  DOutMin=[]  DOutMax=[]  NOutMin=[]  NOutMax=[]  bOutMin=[]  bOutMax=[]  cOutMin=[]  cOutMax=[]  SumOutMin=[]  SumOutMax=[]  SaturationOutMin=[]  SaturationOutMax=[]  PParamMin=[]  PParamMax=[]  IParamMin=[]  IParamMax=[]  DParamMin=[]  DParamMax=[]  NParamMin=[]  NParamMax=[]  bParamMin=[]  bParamMax=[]  cParamMin=[]  cParamMax=[]  KbParamMin=[]  KbParamMax=[]  KtParamMin=[]  KtParamMax=[]  KbOutMin=[]  KbOutMax=[]  KtOutMin=[]  KtOutMax=[]  IntegratorOutMin=[]  IntegratorOutMax=[]  FilterOutMin=[]  FilterOutMax=[]  SumI1OutMin=[]  SumI1OutMax=[]  SumI2OutMin=[]  SumI2OutMax=[]  SumI3OutMin=[]  SumI3OutMax=[]  SumI4OutMin=[]  SumI4OutMax=[]  SumDOutMin=[]  SumDOutMax=[]  Sum1OutMin=[]  Sum1OutMax=[]  Sum2OutMin=[]  Sum2OutMax=[]  Sum3OutMin=[]  Sum3OutMax=[]  DifferentiatorOutMin=[]  DifferentiatorOutMax=[]  FilterDiffOutCoefMin=[]  FilterDiffOutCoefMax=[]  ReciprocalOutMin=[]  ReciprocalOutMax=[]  SumDenOutMin=[]  SumDenOutMax=[]  SumNumOutMin=[]  SumNumOutMax=[]  DivideOutMin=[]  DivideOutMax=[]  UdiffTsProdOutMin=[]  UdiffTsProdOutMax=[]  NTsProdOutMin=[]  NTsProdOutMax=[]  UintegralTsProdOutMin=[]  UintegralTsProdOutMax=[]  UngainTsProdOutMin=[]  UngainTsProdOutMax=[]  ClampingZeroOutDataTypeStr=Inherit: Inherit via back propagation  ClampingZeroOutMin=[]  ClampingZeroOutMax=[]  FilterDenConstantOutDataTypeStr=Inherit: Inherit via back propagation  FilterDenConstantOutMin=[]  FilterDenConstantOutMax=[]  PCopyOutDataTypeStr=Inherit: Inherit via back propagation  PCopyOutMin=[]  PCopyOutMax=[]  NCopyOutDataTypeStr=Inherit: Inherit via back propagation  NCopyOutMin=[]  NCopyOutMax=[]  IntegratorContinuousStateAttributes=''  IntegratorStateMustResolveToSignalObject=off  IntegratorRTWStateStorageClass=Auto  FilterContinuousStateAttributes=''  FilterStateMustResolveToSignalObject=off  FilterRTWStateStorageClass=Auto  ParallelPVariant=InternalParameters  IdealPVariant=Disabled  IVariant=InternalParameters  DVariant=InternalParameters  bVariant=InternalParameters  cVariant=InternalParameters  IntegratorVariant=Continuous  SatVariant=Enabled  AWVariant=Passthrough  PCopyVariant=Disabled  TRVariant=Disabled  FdbkBlocksVariant=Forward  IdealPFdbkVariant=Disabled  SatFdbkVariant=Disabled  DerivativeFilterVariant=ContFilter  NVariant=InternalParameters  NCopyVariant=Disabled  FilterICVariant=InternalICsFilter  IntegratorICVariant=InternalICs  ExternalResetVariant=Disabled  TRSumVariant=Passthrough  SumFdbkVariant=Disabled  SumVariant=Sum_PID  TsampFilterVariant=InternalTs  TsampNgainVariant=Passthrough  TsampIntegralVariant=Disabled_SignalSpec  ExternalSaturationOutDataTypeStr=Inherit: Same as second input
  Out1 : Outport
  " " : Outport  Port=2
  wires:
  PID Controller (2DOF)/1 -> Out1/1
  States/1 -> " "/1, MATLAB Function/1(X)
  MATLAB Function/1(Aircraft_Airspeed) -> PID Controller (2DOF)/2
  Reference/1 -> PID Controller (2DOF)/1

== system VectorTrackingSim/Control/Subsystem4 ==
  Reference : Inport
  States : Inport  Port=2
  Display : Display
  Display1 : Display
  Display2 : Display
  PID Controller (2DOF) : slpidlib/PID Controller (2DOF)  Controller=PID  Form=Parallel  TimeDomain=Continuous-time  UseExternalTs=off  SampleTime=-1  IntegratorMethod=Forward Euler  FilterMethod=Forward Euler  ControllerParametersSource=internal  P=0  I=1  UseKiTs=off  D=0  N=100  UseFilter=on  b=1  c=1  TunerSelectOption=Transfer Function Based (PID Tuner App)  InitialConditionSource=internal  InitialConditionForIntegrator=0  InitialConditionForFilter=0  DifferentiatorICPrevScaledInput=0  ExternalReset=none  TrackingMode=off  Kt=1  LimitOutput=on  SatLimitsSource=internal  UpperSaturationLimit=1  LowerSaturationLimit=0  LinearizeAsGain=on  AntiWindupMode=none  Kb=1  LimitIntegrator=off  UpperIntegratorSaturationLimit=inf  LowerIntegratorSaturationLimit=-inf  POutMin=[]  POutMax=[]  IOutMin=[]  IOutMax=[]  DOutMin=[]  DOutMax=[]  NOutMin=[]  NOutMax=[]  bOutMin=[]  bOutMax=[]  cOutMin=[]  cOutMax=[]  SumOutMin=[]  SumOutMax=[]  SaturationOutMin=[]  SaturationOutMax=[]  PParamMin=[]  PParamMax=[]  IParamMin=[]  IParamMax=[]  DParamMin=[]  DParamMax=[]  NParamMin=[]  NParamMax=[]  bParamMin=[]  bParamMax=[]  cParamMin=[]  cParamMax=[]  KbParamMin=[]  KbParamMax=[]  KtParamMin=[]  KtParamMax=[]  KbOutMin=[]  KbOutMax=[]  KtOutMin=[]  KtOutMax=[]  IntegratorOutMin=[]  IntegratorOutMax=[]  FilterOutMin=[]  FilterOutMax=[]  SumI1OutMin=[]  SumI1OutMax=[]  SumI2OutMin=[]  SumI2OutMax=[]  SumI3OutMin=[]  SumI3OutMax=[]  SumI4OutMin=[]  SumI4OutMax=[]  SumDOutMin=[]  SumDOutMax=[]  Sum1OutMin=[]  Sum1OutMax=[]  Sum2OutMin=[]  Sum2OutMax=[]  Sum3OutMin=[]  Sum3OutMax=[]  DifferentiatorOutMin=[]  DifferentiatorOutMax=[]  FilterDiffOutCoefMin=[]  FilterDiffOutCoefMax=[]  ReciprocalOutMin=[]  ReciprocalOutMax=[]  SumDenOutMin=[]  SumDenOutMax=[]  SumNumOutMin=[]  SumNumOutMax=[]  DivideOutMin=[]  DivideOutMax=[]  UdiffTsProdOutMin=[]  UdiffTsProdOutMax=[]  NTsProdOutMin=[]  NTsProdOutMax=[]  UintegralTsProdOutMin=[]  UintegralTsProdOutMax=[]  UngainTsProdOutMin=[]  UngainTsProdOutMax=[]  ClampingZeroOutDataTypeStr=Inherit: Inherit via back propagation  ClampingZeroOutMin=[]  ClampingZeroOutMax=[]  FilterDenConstantOutDataTypeStr=Inherit: Inherit via back propagation  FilterDenConstantOutMin=[]  FilterDenConstantOutMax=[]  PCopyOutDataTypeStr=Inherit: Inherit via back propagation  PCopyOutMin=[]  PCopyOutMax=[]  NCopyOutDataTypeStr=Inherit: Inherit via back propagation  NCopyOutMin=[]  NCopyOutMax=[]  IntegratorContinuousStateAttributes=''  IntegratorStateMustResolveToSignalObject=off  IntegratorRTWStateStorageClass=Auto  FilterContinuousStateAttributes=''  FilterStateMustResolveToSignalObject=off  FilterRTWStateStorageClass=Auto  ParallelPVariant=InternalParameters  IdealPVariant=Disabled  IVariant=InternalParameters  DVariant=InternalParameters  bVariant=InternalParameters  cVariant=InternalParameters  IntegratorVariant=Continuous  SatVariant=Enabled  AWVariant=Passthrough  PCopyVariant=Disabled  TRVariant=Disabled  FdbkBlocksVariant=Forward  IdealPFdbkVariant=Disabled  SatFdbkVariant=Disabled  DerivativeFilterVariant=ContFilter  NVariant=InternalParameters  NCopyVariant=Disabled  FilterICVariant=InternalICsFilter  IntegratorICVariant=InternalICs  ExternalResetVariant=Disabled  TRSumVariant=Passthrough  SumFdbkVariant=Disabled  SumVariant=Sum_PID  TsampFilterVariant=InternalTs  TsampNgainVariant=Passthrough  TsampIntegralVariant=Disabled_SignalSpec  ExternalSaturationOutDataTypeStr=Inherit: Same as second input
  Out1 : Outport
  " " : Outport  Port=2
  wires:
  PID Controller (2DOF)/1 -> Display2/1, Out1/1
  [truepropEff] -> Display/1, PID Controller (2DOF)/2
  Reference/1 -> Display1/1, PID Controller (2DOF)/1
  States/1 -> " "/1

== system VectorTrackingSim/Control/Subsystem5 ==
  Reference : Inport
  States : Inport  Port=2
  Out1 : Outport
  " " : Outport  Port=2
  wires:
  Reference/1 -> Out1/1
  States/1 -> " "/1

== system VectorTrackingSim/Control/Subsystem6 ==
  Reference : Inport
  States : Inport  Port=2
  Out1 : Outport
  " " : Outport  Port=2
  wires:
  Reference/1 -> Out1/1
  States/1 -> " "/1

== system VectorTrackingSim/Control/Subsystem7 ==
  Reference : Inport
  States : Inport  Port=2
  Out1 : Outport
  " " : Outport  Port=2
  wires:
  Reference/1 -> Out1/1
  States/1 -> " "/1

== system VectorTrackingSim/Control/Subsystem8 ==
  Reference : Inport
  States : Inport  Port=2
  Out1 : Outport
  " " : Outport  Port=2
  wires:
  Reference/1 -> Out1/1
  States/1 -> " "/1

== system VectorTrackingSim/Control/Subsystem9 ==
  Reference : Inport
  States : Inport  Port=2
  Out1 : Outport
  " " : Outport  Port=2
  wires:
  States/1 -> " "/1
  Reference/1 -> Out1/1

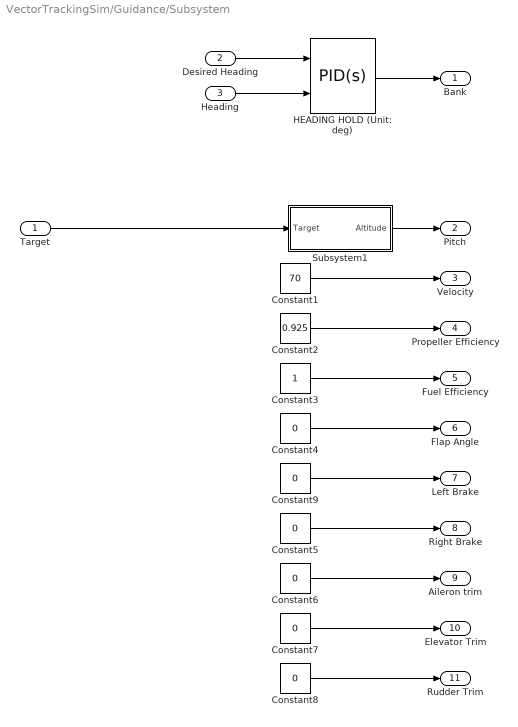
== system VectorTrackingSim/Guidance/Subsystem ==
  Target : Inport
  Desired Heading : Inport  Port=2
  Heading : Inport  Port=3
  Constant1 : Constant  Value=70
  Constant2 : Constant  Value=0.925
  Constant3 : Constant
  Constant{4..9} (6 alike) : Constant  Value=0
  HEADING HOLD (Unit: deg) : slpidlib/PID Controller (2DOF)  Controller=PID  Form=Parallel  TimeDomain=Continuous-time  UseExternalTs=off  SampleTime=-1  IntegratorMethod=Forward Euler  FilterMethod=Forward Euler  ControllerParametersSource=internal  P=1  I=0.001  UseKiTs=off  D=0  N=100  UseFilter=on  b=1  c=0  TunerSelectOption=Transfer Function Based (PID Tuner App)  InitialConditionSource=internal  InitialConditionForIntegrator=0  InitialConditionForFilter=0  DifferentiatorICPrevScaledInput=0  ExternalReset=none  TrackingMode=off  Kt=1  LimitOutput=on  SatLimitsSource=internal  UpperSaturationLimit=30  LowerSaturationLimit=-30  LinearizeAsGain=on  AntiWindupMode=clamping  Kb=1  LimitIntegrator=off  UpperIntegratorSaturationLimit=inf  LowerIntegratorSaturationLimit=-inf  POutMin=[]  POutMax=[]  IOutMin=[]  IOutMax=[]  DOutMin=[]  DOutMax=[]  NOutMin=[]  NOutMax=[]  bOutMin=[]  bOutMax=[]  cOutMin=[]  cOutMax=[]  SumOutMin=[]  SumOutMax=[]  SaturationOutMin=[]  SaturationOutMax=[]  PParamMin=[]  PParamMax=[]  IParamMin=[]  IParamMax=[]  DParamMin=[]  DParamMax=[]  NParamMin=[]  NParamMax=[]  bParamMin=[]  bParamMax=[]  cParamMin=[]  cParamMax=[]  KbParamMin=[]  KbParamMax=[]  KtParamMin=[]  KtParamMax=[]  KbOutMin=[]  KbOutMax=[]  KtOutMin=[]  KtOutMax=[]  IntegratorOutMin=[]  IntegratorOutMax=[]  FilterOutMin=[]  FilterOutMax=[]  SumI1OutMin=[]  SumI1OutMax=[]  SumI2OutMin=[]  SumI2OutMax=[]  SumI3OutMin=[]  SumI3OutMax=[]  SumI4OutMin=[]  SumI4OutMax=[]  SumDOutMin=[]  SumDOutMax=[]  Sum1OutMin=[]  Sum1OutMax=[]  Sum2OutMin=[]  Sum2OutMax=[]  Sum3OutMin=[]  Sum3OutMax=[]  DifferentiatorOutMin=[]  DifferentiatorOutMax=[]  FilterDiffOutCoefMin=[]  FilterDiffOutCoefMax=[]  ReciprocalOutMin=[]  ReciprocalOutMax=[]  SumDenOutMin=[]  SumDenOutMax=[]  SumNumOutMin=[]  SumNumOutMax=[]  DivideOutMin=[]  DivideOutMax=[]  UdiffTsProdOutMin=[]  UdiffTsProdOutMax=[]  NTsProdOutMin=[]  NTsProdOutMax=[]  UintegralTsProdOutMin=[]  UintegralTsProdOutMax=[]  UngainTsProdOutMin=[]  UngainTsProdOutMax=[]  ClampingZeroOutDataTypeStr=Inherit: Inherit via back propagation  ClampingZeroOutMin=[]  ClampingZeroOutMax=[]  FilterDenConstantOutDataTypeStr=Inherit: Inherit via back propagation  FilterDenConstantOutMin=[]  FilterDenConstantOutMax=[]  PCopyOutDataTypeStr=Inherit: Inherit via back propagation  PCopyOutMin=[]  PCopyOutMax=[]  NCopyOutDataTypeStr=Inherit: Inherit via back propagation  NCopyOutMin=[]  NCopyOutMax=[]  IntegratorContinuousStateAttributes=''  IntegratorStateMustResolveToSignalObject=off  IntegratorRTWStateStorageClass=Auto  FilterContinuousStateAttributes=''  FilterStateMustResolveToSignalObject=off  FilterRTWStateStorageClass=Auto  ParallelPVariant=InternalParameters  IdealPVariant=Disabled  IVariant=InternalParameters  DVariant=InternalParameters  bVariant=InternalParameters  cVariant=InternalParameters  IntegratorVariant=Continuous  SatVariant=Enabled  AWVariant=ContClampingParallel  PCopyVariant=Disabled  TRVariant=Disabled  FdbkBlocksVariant=Forward  IdealPFdbkVariant=Disabled  SatFdbkVariant=Disabled  DerivativeFilterVariant=ContFilter  NVariant=InternalParameters  NCopyVariant=Disabled  FilterICVariant=InternalICsFilter  IntegratorICVariant=InternalICs  ExternalResetVariant=Disabled  TRSumVariant=Passthrough  SumFdbkVariant=Disabled  SumVariant=Sum_PID  TsampFilterVariant=InternalTs  TsampNgainVariant=Passthrough  TsampIntegralVariant=Disabled_SignalSpec  ExternalSaturationOutDataTypeStr=Inherit: Same as second input
  Subsystem1 : Subsystem
  Bank : Outport
  Pitch : Outport  Port=2
  Velocity : Outport  Port=3
  Propeller Efficiency : Outport  Port=4
  Fuel Efficiency : Outport  Port=5
  Flap Angle : Outport  Port=6
  Left Brake : Outport  Port=7
  Right Brake : Outport  Port=8
  Aileron trim : Outport  Port=9
  Elevator Trim : Outport  Port=10
  Rudder Trim : Outport  Port=11
  wires:
  Subsystem1/1(Altitude) -> Pitch/1
  Constant1/1 -> Velocity/1
  Constant2/1 -> Propeller Efficiency/1
  Constant3/1 -> Fuel Efficiency/1
  Constant4/1 -> Flap Angle/1
  Constant9/1 -> Left Brake/1
  Constant5/1 -> Right Brake/1
  Constant6/1 -> Aileron trim/1
  Constant7/1 -> Elevator Trim/1
  Constant8/1 -> Rudder Trim/1
  Desired Heading/1 -> HEADING HOLD (Unit: deg)/1
  Target/1 -> Subsystem1/1(Target)
  HEADING HOLD (Unit: deg)/1 -> Bank/1
  Heading/1 -> HEADING HOLD (Unit: deg)/2

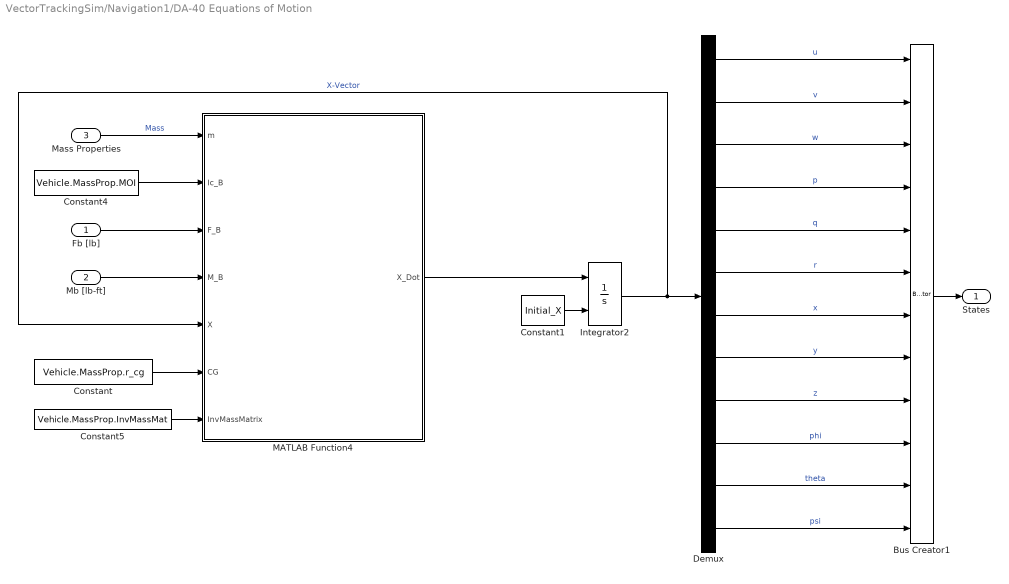
== system VectorTrackingSim/Navigation1/DA-40 Equations of Motion ==
  Fb [lb] : Inport
  Mb [lb-ft] : Inport  Port=2
  Mass Properties : Inport  Port=3
  Bus Creator1 : BusCreator  Inputs=12
  Constant : Constant  Value=Vehicle.MassProp.r_cg
  Constant1 : Constant  Value=Initial_X
  Constant4 : Constant  Value=Vehicle.MassProp.MOI  VectorParams1D=off
  Constant5 : Constant  Value=Vehicle.MassProp.InvMassMat
  Demux : Demux  Outputs=12
  Integrator2 : Integrator  InitialConditionSource=external
  MATLAB Function4 : MATLAB Function  TreatAsAtomicUnit=on
  States : Outport
  wires:
  Mb [lb-ft]/1 -> MATLAB Function4/4(M_B)
  Fb [lb]/1 -> MATLAB Function4/3(F_B)
  Mass Properties/1 -> MATLAB Function4/1(m)  "Mass"
  Constant4/1 -> MATLAB Function4/2(Ic_B)
  Constant1/1 -> Integrator2/2
  Integrator2/1 -> MATLAB Function4/5(X), Demux/1  "X-Vector"
  Constant/1 -> MATLAB Function4/6(CG)
  Constant5/1 -> MATLAB Function4/7(InvMassMatrix)
  Demux/1 -> Bus Creator1/1  "u"
  Demux/2 -> Bus Creator1/2  "v"
  Demux/3 -> Bus Creator1/3  "w"
  Demux/4 -> Bus Creator1/4  "p"
  Demux/5 -> Bus Creator1/5  "q"
  Demux/6 -> Bus Creator1/6  "r"
  Demux/7 -> Bus Creator1/7  "x"
  Demux/8 -> Bus Creator1/8  "y"
  Demux/9 -> Bus Creator1/9  "z"
  Demux/10 -> Bus Creator1/10  "phi"
  Demux/11 -> Bus Creator1/11  "theta"
  Demux/12 -> Bus Creator1/12  "psi"
  MATLAB Function4/1(X_Dot) -> Integrator2/1
  Bus Creator1/1 -> States/1
